simulink model "MyCtrler"  (R2025b)
settings: Solver=ode14x  StartTime=0.0  StopTime=10.0  FixedStep=Ts_local  RelTol=1e-3
values from neighbouring files (symbols this model uses):
  Ts_ctrl = 0.02    [ctrlSys.sldd]
settings Model: DataDictionary=ctrlSys.sldd  Creator=LYG  LastModifiedBy=LYG

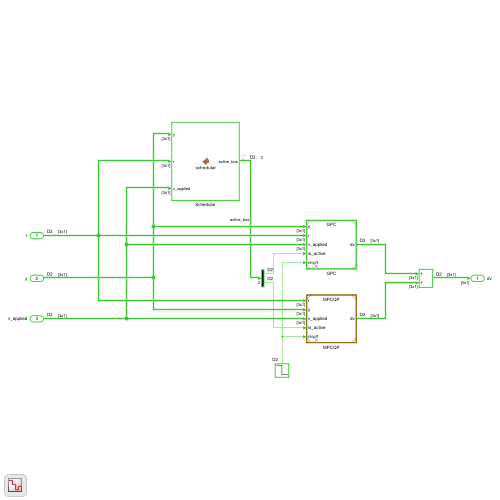
[thumbnail: Simulink's stored preview of the top-level diagram]
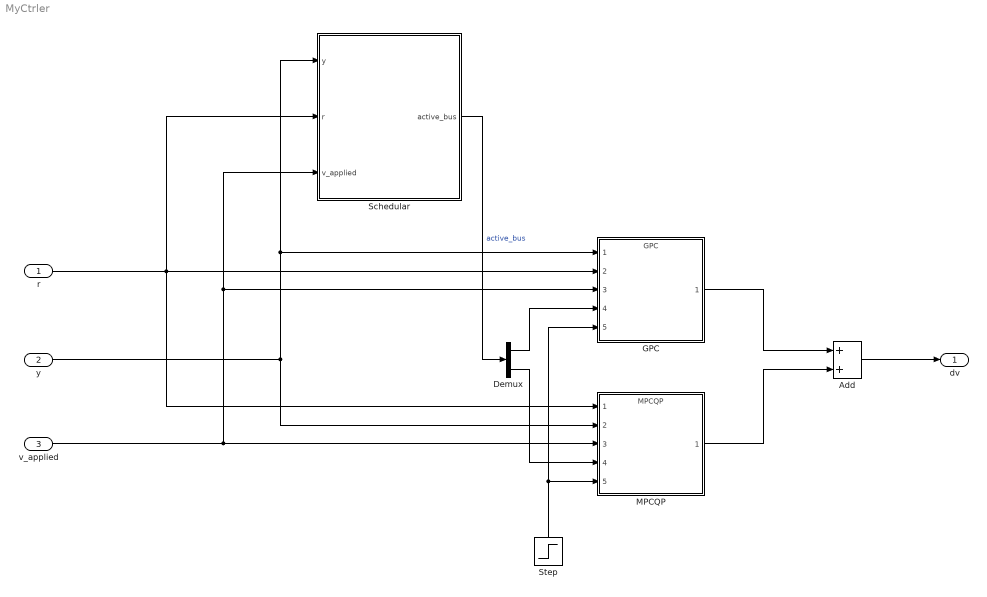
== system MyCtrler ==
  r : Inport
  y : Inport  Port=2
  v_applied : Inport  Port=3
  Add : Sum
  Demux : Demux  Outputs=2
  GPC : ModelReference  ModelNameDialog=GPC.slx  SimulationMode=Normal  ModelReferenceVersion=1.264
  MPCQP : ModelReference  ModelNameDialog=MPCQP.slx  SimulationMode=Normal  ModelReferenceVersion=1.56
  Schedular : MATLAB Function  TreatAsAtomicUnit=on  SystemSampleTime=Ts_ctrl
  Step : Step  Time=0.1  Before=1  After=0  SampleTime=Ts_ctrl
  dv : Outport
  wires:
  v_applied/1 -> Schedular/3(v_applied), GPC/3, MPCQP/3
  y/1 -> MPCQP/2, Schedular/1(y), GPC/1
  r/1 -> Schedular/2(r), MPCQP/1, GPC/2
  Add/1 -> dv/1
  MPCQP/1 -> Add/2
  GPC/1 -> Add/1
  Step/1 -> GPC/5, MPCQP/5
  Demux/2 -> MPCQP/4
  Demux/1 -> GPC/4
  Schedular/1(active_bus) -> Demux/1  "active_bus"

== matlab function MyCtrler/Schedular ==
  data: y input size=[3 1]; r input size=[3 1]; active_bus output boolean; v_applied input size=[3 1]
function active_bus = schedular(y, r, v_applied)

    persistent r_prev state cnt;

    % Define states
    REF_CHANGE = 1;
    STABLE     = 2;
    BRIDGE     = 3;

    % Tolerance for floating-point comparison
    tol = 1e-2;

    % Initialization
    if isempty(r_prev)
        r_prev = zeros(size(r));
    end

    if isempty(state)
        state = REF_CHANGE;
    end

    if isempty(cnt)
        cnt = 0;
    end

    % -------- State Transition Logic --------
    if state == STABLE && any(abs(r - r_prev) > tol)
        % Reference changed
        state = REF_CHANGE;

    elseif state == REF_CHANGE && any(abs(y - r) > tol)
        % Any element not equal → still in RefChange
        state = REF_CHANGE;

    elseif (state == REF_CHANGE || state == BRIDGE) && (cnt <= 250)
        state = BRIDGE;

    else
        % All elements match → Stable
        state = STABLE;
    end

    % -------- Output Logic --------
    switch state
        case REF_CHANGE
            active_bus = [0; 1];
        case STABLE
            cnt = 0;
            active_bus = [1; 0];
        case BRIDGE
            cnt = cnt + 1;
            active_bus = [0; 1];
        otherwise
            active_bus = [0; 0];
    end

    % Update previous reference
    r_prev = r;

    % Logical output
    active_bus = logical(active_bus);
end
